simulink model "Raider_walk"  (R2016a)
settings: Solver=FixedStepAuto  StartTime=0.0  StopTime=inf  FixedStep=0.01  RelTol=1e-3
model workspace (MAT data in the model file):
  SL_ROS_VariableLengthArrays_MaxSizes.CommonInfo.ArrayTruncateAction = 'EmitWarning'
  SL_ROS_VariableLengthArrays_MaxSizes.MsgTypeMap = containers.Map
  SL_ROS_VariableLengthArrays_MaxSizes.MsgTypeMap.serialization.keys = {'sensor_msgs/JointState'}
  SL_ROS_VariableLengthArrays_MaxSizes.MsgTypeMap.serialization.values{1}(1).PropertyName = 'Name'
  SL_ROS_VariableLengthArrays_MaxSizes.MsgTypeMap.serialization.values{1}(1).DataType = 'std_msgs/String'
  SL_ROS_VariableLengthArrays_MaxSizes.MsgTypeMap.serialization.values{1}(1).MaxLength = 20
  SL_ROS_VariableLengthArrays_MaxSizes.MsgTypeMap.serialization.values{1}(2).PropertyName = 'Position'
  SL_ROS_VariableLengthArrays_MaxSizes.MsgTypeMap.serialization.values{1}(2).DataType = 'double'
  SL_ROS_VariableLengthArrays_MaxSizes.MsgTypeMap.serialization.values{1}(2).MaxLength = 128
  SL_ROS_VariableLengthArrays_MaxSizes.MsgTypeMap.serialization.values{1}(3).PropertyName = 'Velocity'
  SL_ROS_VariableLengthArrays_MaxSizes.MsgTypeMap.serialization.values{1}(3).DataType = 'double'
  SL_ROS_VariableLengthArrays_MaxSizes.MsgTypeMap.serialization.values{1}(3).MaxLength = 128
  SL_ROS_VariableLengthArrays_MaxSizes.MsgTypeMap.serialization.values{1}(4).PropertyName = 'Effort'
  SL_ROS_VariableLengthArrays_MaxSizes.MsgTypeMap.serialization.values{1}(4).DataType = 'double'
  SL_ROS_VariableLengthArrays_MaxSizes.MsgTypeMap.serialization.values{1}(4).MaxLength = 128
  SL_ROS_VariableLengthArrays_MaxSizes.MsgTypeMap.serialization.uniformity = 0
  SL_ROS_VariableLengthArrays_MaxSizes.MsgTypeMap.serialization.keyType = 'char'
  SL_ROS_VariableLengthArrays_MaxSizes.MsgTypeMap.serialization.valueType = 'any'
  currentPosition = Simulink.Signal
  currentPosition.DataType = 'double'
  currentPosition.Dimensions = [1 20]
  currentPosition.DimensionsMode = 'auto'
  currentPosition.Complexity = 'real'
  currentPosition.SampleTime = -1
  currentPosition.SamplingMode = 'auto'
  currentPosition.InitialValue = '[0 0 0 0 0 0 0 0 0 0 0 0 0 0 0 0 0 0 0 0]'
  targetPosition = Simulink.Signal
  targetPosition.DataType = 'double'
  targetPosition.Dimensions = [1 20]
  targetPosition.DimensionsMode = 'auto'
  targetPosition.Complexity = 'real'
  targetPosition.SampleTime = -1
  targetPosition.SamplingMode = 'auto'
  targetPosition.InitialValue = '[0 0 0 0 0 0 0 0 0 0 0 0 0 0 0 0 0 0 0 0]'
libraries: robotlib x81
(part 1 of 2)
settings Model: Creator=xavidz  LastModifiedBy=xavidz
settings OptimizationCC: OptimizeModelRefInitCode=on  LifeSpan=1  MaxStackSize=64
settings HardwareCC: ProdBitPerLong=64  ProdHWDeviceType=Intel->x86-64 (Linux 64)
settings RTWCC: SystemTargetFile=ert.tlc  HardwareBoard=Robot Operating System (ROS)  TemplateMakefile=ert_default_tmf  GenerateReport=on  Toolchain=Catkin  IncludeHyperlinkInReport=on  LaunchReport=on  TargetLang=C++  GenerateTraceInfo=on  GenerateTraceReport=on  GenerateTraceReportSl=on  GenerateTraceReportSf=on  GenerateTraceReportEml=on
settings CodeAppCC: ForceParamTrailComments=on  IgnoreCustomStorageClasses=off  OperatorAnnotations=on  SimulinkDataObjDesc=on  SFDataObjDesc=on  MATLABFcnDesc=on  InsertBlockDesc=on  MATLABSourceComments=on

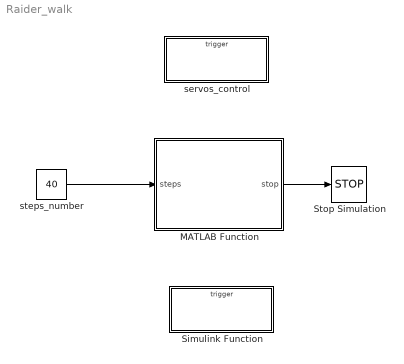
== system Raider_walk ==
  MATLAB Function : MATLAB Function  TreatAsAtomicUnit=on
  Simulink Function : Subsystem  TreatAsAtomicUnit=on
  Stop Simulation : Stop
  servos_control : Subsystem  TreatAsAtomicUnit=on
  "steps_number " : Constant  Value=40  OutDataTypeStr=uint8
  wires:
  MATLAB Function/1(stop) -> Stop Simulation/1
  "steps_number "/1 -> MATLAB Function/1(steps)

== system Raider_walk/Simulink Function ==
  delay : TriggerPort  TriggerType=function-call  IsSimulinkFunction=on  FunctionName=delay  VariantControl=Variant
  MATLAB Function : MATLAB Function  TreatAsAtomicUnit=on
  Simulink Function4 : Subsystem  TreatAsAtomicUnit=on
  t : ArgIn  DisableCoverage=on  ArgumentName=t
  wires:
  t/1 -> MATLAB Function/1(t)

== system Raider_walk/servos_control ==
  move : TriggerPort  TriggerType=function-call  IsSimulinkFunction=on  FunctionName=move  VariantControl=Variant
  MATLAB Function : MATLAB Function  TreatAsAtomicUnit=on
  Simulink Function1 : Subsystem  TreatAsAtomicUnit=on
  Simulink Function2 : Subsystem  TreatAsAtomicUnit=on
  t : ArgIn  ArgumentName=t
  wires:
  t/1 -> MATLAB Function/1(t)

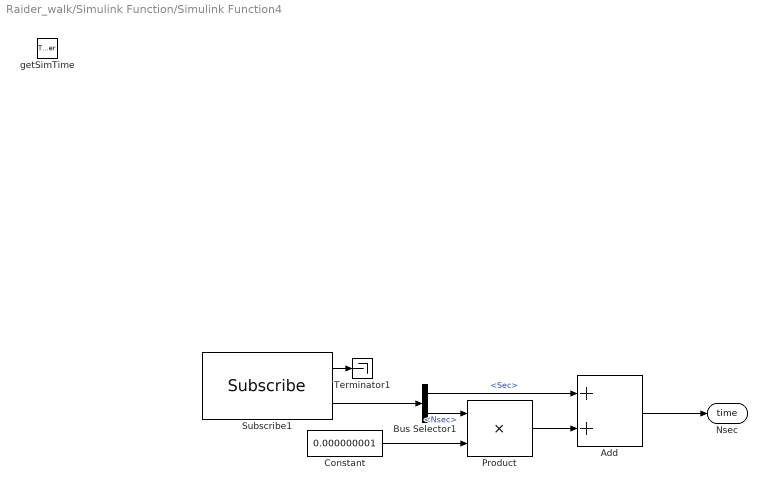
== system Raider_walk/Simulink Function/Simulink Function4 ==
  getSimTime : TriggerPort  TriggerType=function-call  IsSimulinkFunction=on  FunctionName=getSimTime  VariantControl=Variant
  Add : Sum
  Bus Selector1 : BusSelector  OutputSignals=Clock_.Sec,Clock_.Nsec
  Constant : Constant  Value=0.000000001
  Product : Product
  Subscribe1 : robotlib/Subscribe  SourceLibraryInfo=This block requires Robotics System Toolbox  topicSource=Select from ROS network  topic=/clock  messageType=rosgraph_msgs/Clock  sampleTime=-1  messageQueueLength=1
  Terminator1 : Terminator
  Nsec : ArgOut  ArgumentName=time
  wires:
  Subscribe1/2 -> Bus Selector1/1
  Bus Selector1/2 -> Product/1  "<Nsec>"
  Constant/1 -> Product/2
  Bus Selector1/1 -> Add/1  "<Sec>"
  Product/1 -> Add/2
  Add/1 -> Nsec/1
  Subscribe1/1 -> Terminator1/1

== system Raider_walk/servos_control/Simulink Function1 ==
  publishPosition : TriggerPort  TriggerType=function-call  IsSimulinkFunction=on  FunctionName=publishPosition  VariantControl=Variant
  Position_Publishers : Subsystem
  Switch Case : SwitchCase  CaseConditions={1,2,3,4,5,6,7,8,9,10,11,12,13,14,15,16,17,18,19,20}  ShowDefaultCase=off
  joint : ArgIn  DisableCoverage=on  ArgumentName=joint
  pos : ArgIn  Port=2  ArgumentName=pos
  wires:
  joint/1 -> Switch Case/1
  Switch Case/1 -> Position_Publishers/1(In1)
  Switch Case/2 -> Position_Publishers/2(In2)
  Switch Case/3 -> Position_Publishers/3(In3)
  Switch Case/4 -> Position_Publishers/4(In4)
  Switch Case/5 -> Position_Publishers/5(In5)
  Switch Case/6 -> Position_Publishers/6(In6)
  pos/1 -> Position_Publishers/21("In21 ")
  Switch Case/20 -> Position_Publishers/20(In20)
  Switch Case/19 -> Position_Publishers/19(In19)
  Switch Case/18 -> Position_Publishers/18(In18)
  Switch Case/16 -> Position_Publishers/16(In16)
  Switch Case/17 -> Position_Publishers/17(In17)
  Switch Case/15 -> Position_Publishers/15(In15)
  Switch Case/14 -> Position_Publishers/14(In14)
  Switch Case/13 -> Position_Publishers/13(In13)
  Switch Case/12 -> Position_Publishers/12(In12)
  Switch Case/11 -> Position_Publishers/11(In11)
  Switch Case/10 -> Position_Publishers/10(In10)
  Switch Case/9 -> Position_Publishers/9(In9)
  Switch Case/8 -> Position_Publishers/8(In8)
  Switch Case/7 -> Position_Publishers/7(In7)

== system Raider_walk/servos_control/Simulink Function2 ==
  publishVelocity : TriggerPort  TriggerType=function-call  IsSimulinkFunction=on  FunctionName=publishVelocity  VariantControl=Variant
  Switch Case : SwitchCase  CaseConditions={1,2,3,4,5,6,7,8,9,10,11,12,13,14,15,16,17,18,19,20}  ShowDefaultCase=off
  Velocity_Publishers : Subsystem
  joint : ArgIn  DisableCoverage=on  ArgumentName=joint
  vel : ArgIn  Port=2  ArgumentName=vel
  wires:
  joint/1 -> Switch Case/1
  Switch Case/1 -> Velocity_Publishers/1(In1)
  Switch Case/2 -> Velocity_Publishers/2(In2)
  Switch Case/3 -> Velocity_Publishers/3(In3)
  Switch Case/4 -> Velocity_Publishers/4(In4)
  Switch Case/5 -> Velocity_Publishers/5(In5)
  Switch Case/6 -> Velocity_Publishers/6(In6)
  vel/1 -> Velocity_Publishers/21("In21 ")
  Switch Case/20 -> Velocity_Publishers/20(In20)
  Switch Case/19 -> Velocity_Publishers/19(In19)
  Switch Case/18 -> Velocity_Publishers/18(In18)
  Switch Case/16 -> Velocity_Publishers/16(In16)
  Switch Case/17 -> Velocity_Publishers/17(In17)
  Switch Case/15 -> Velocity_Publishers/15(In15)
  Switch Case/14 -> Velocity_Publishers/14(In14)
  Switch Case/13 -> Velocity_Publishers/13(In13)
  Switch Case/12 -> Velocity_Publishers/12(In12)
  Switch Case/11 -> Velocity_Publishers/11(In11)
  Switch Case/10 -> Velocity_Publishers/10(In10)
  Switch Case/9 -> Velocity_Publishers/9(In9)
  Switch Case/8 -> Velocity_Publishers/8(In8)
  Switch Case/7 -> Velocity_Publishers/7(In7)

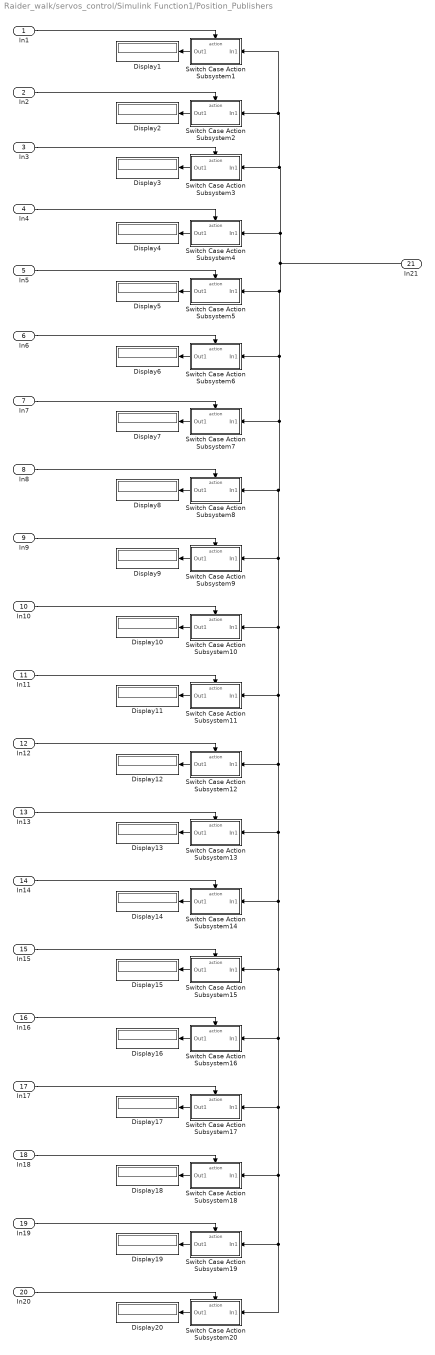
== system Raider_walk/servos_control/Simulink Function1/Position_Publishers ==
  In1 : Inport
  In2 : Inport  Port=2
  In3 : Inport  Port=3
  In4 : Inport  Port=4
  In5 : Inport  Port=5
  In6 : Inport  Port=6
  In7 : Inport  Port=7
  In8 : Inport  Port=8
  In9 : Inport  Port=9
  In10 : Inport  Port=10
  In11 : Inport  Port=11
  In12 : Inport  Port=12
  In13 : Inport  Port=13
  In14 : Inport  Port=14
  In15 : Inport  Port=15
  In16 : Inport  Port=16
  In17 : Inport  Port=17
  In18 : Inport  Port=18
  In19 : Inport  Port=19
  In20 : Inport  Port=20
  "In21 " : Inport  Port=21
  Display{1..20} (20 alike) : Display
  "Switch Case Action Subsystem1 " : Subsystem  TreatAsAtomicUnit=on
  Switch Case Action Subsystem10 : Subsystem  TreatAsAtomicUnit=on
  Switch Case Action Subsystem11 : Subsystem  TreatAsAtomicUnit=on
  Switch Case Action Subsystem12 : Subsystem  TreatAsAtomicUnit=on
  Switch Case Action Subsystem13 : Subsystem  TreatAsAtomicUnit=on
  Switch Case Action Subsystem14 : Subsystem  TreatAsAtomicUnit=on
  Switch Case Action Subsystem15 : Subsystem  TreatAsAtomicUnit=on
  Switch Case Action Subsystem16 : Subsystem  TreatAsAtomicUnit=on
  Switch Case Action Subsystem17 : Subsystem  TreatAsAtomicUnit=on
  Switch Case Action Subsystem18 : Subsystem  TreatAsAtomicUnit=on
  Switch Case Action Subsystem19 : Subsystem  TreatAsAtomicUnit=on
  "Switch Case Action Subsystem2 " : Subsystem  TreatAsAtomicUnit=on
  Switch Case Action Subsystem20 : Subsystem  TreatAsAtomicUnit=on
  "Switch Case Action Subsystem3 " : Subsystem  TreatAsAtomicUnit=on
  "Switch Case Action Subsystem4 " : Subsystem  TreatAsAtomicUnit=on
  "Switch Case Action Subsystem5 " : Subsystem  TreatAsAtomicUnit=on
  "Switch Case Action Subsystem6 " : Subsystem  TreatAsAtomicUnit=on
  Switch Case Action Subsystem7 : Subsystem  TreatAsAtomicUnit=on
  Switch Case Action Subsystem8 : Subsystem  TreatAsAtomicUnit=on
  Switch Case Action Subsystem9 : Subsystem  TreatAsAtomicUnit=on
  wires:
  "In21 "/1 -> "Switch Case Action Subsystem1 "/1(In1), "Switch Case Action Subsystem2 "/1(In1), "Switch Case Action Subsystem3 "/1(In1), "Switch Case Action Subsystem4 "/1(In1), Switch Case Action Subsystem20/1(In1), Switch Case Action Subsystem19/1(In1), Switch Case Action Subsystem18/1(In1), Switch Case Action Subsystem17/1(In1), Switch Case Action Subsystem16/1(In1), Switch Case Action Subsystem15/1(In1), Switch Case Action Subsystem14/1(In1), Switch Case Action Subsystem13/1(In1), Switch Case Action Subsystem12/1(In1), Switch Case Action Subsystem11/1(In1), Switch Case Action Subsystem10/1(In1), Switch Case Action Subsystem9/1(In1), Switch Case Action Subsystem8/1(In1), Switch Case Action Subsystem7/1(In1), "Switch Case Action Subsystem6 "/1(In1), "Switch Case Action Subsystem5 "/1(In1)
  In1/1 -> "Switch Case Action Subsystem1 "/Action
  In6/1 -> "Switch Case Action Subsystem6 "/Action
  In3/1 -> "Switch Case Action Subsystem3 "/Action
  "Switch Case Action Subsystem5 "/1(Out1) -> Display5/1
  "Switch Case Action Subsystem3 "/1(Out1) -> Display3/1
  "Switch Case Action Subsystem2 "/1(Out1) -> Display2/1
  In4/1 -> "Switch Case Action Subsystem4 "/Action
  "Switch Case Action Subsystem6 "/1(Out1) -> Display6/1
  "Switch Case Action Subsystem1 "/1(Out1) -> Display1/1
  In2/1 -> "Switch Case Action Subsystem2 "/Action
  "Switch Case Action Subsystem4 "/1(Out1) -> Display4/1
  In5/1 -> "Switch Case Action Subsystem5 "/Action
  In7/1 -> Switch Case Action Subsystem7/Action
  Switch Case Action Subsystem7/1(Out1) -> Display7/1
  In8/1 -> Switch Case Action Subsystem8/Action
  Switch Case Action Subsystem8/1(Out1) -> Display8/1
  In9/1 -> Switch Case Action Subsystem9/Action
  Switch Case Action Subsystem9/1(Out1) -> Display9/1
  In10/1 -> Switch Case Action Subsystem10/Action
  Switch Case Action Subsystem10/1(Out1) -> Display10/1
  In11/1 -> Switch Case Action Subsystem11/Action
  Switch Case Action Subsystem11/1(Out1) -> Display11/1
  In12/1 -> Switch Case Action Subsystem12/Action
  Switch Case Action Subsystem12/1(Out1) -> Display12/1
  In13/1 -> Switch Case Action Subsystem13/Action
  Switch Case Action Subsystem13/1(Out1) -> Display13/1
  In14/1 -> Switch Case Action Subsystem14/Action
  Switch Case Action Subsystem14/1(Out1) -> Display14/1
  In15/1 -> Switch Case Action Subsystem15/Action
  Switch Case Action Subsystem15/1(Out1) -> Display15/1
  In16/1 -> Switch Case Action Subsystem16/Action
  Switch Case Action Subsystem16/1(Out1) -> Display16/1
  In17/1 -> Switch Case Action Subsystem17/Action
  Switch Case Action Subsystem17/1(Out1) -> Display17/1
  In18/1 -> Switch Case Action Subsystem18/Action
  Switch Case Action Subsystem18/1(Out1) -> Display18/1
  In19/1 -> Switch Case Action Subsystem19/Action
  Switch Case Action Subsystem19/1(Out1) -> Display19/1
  In20/1 -> Switch Case Action Subsystem20/Action
  Switch Case Action Subsystem20/1(Out1) -> Display20/1

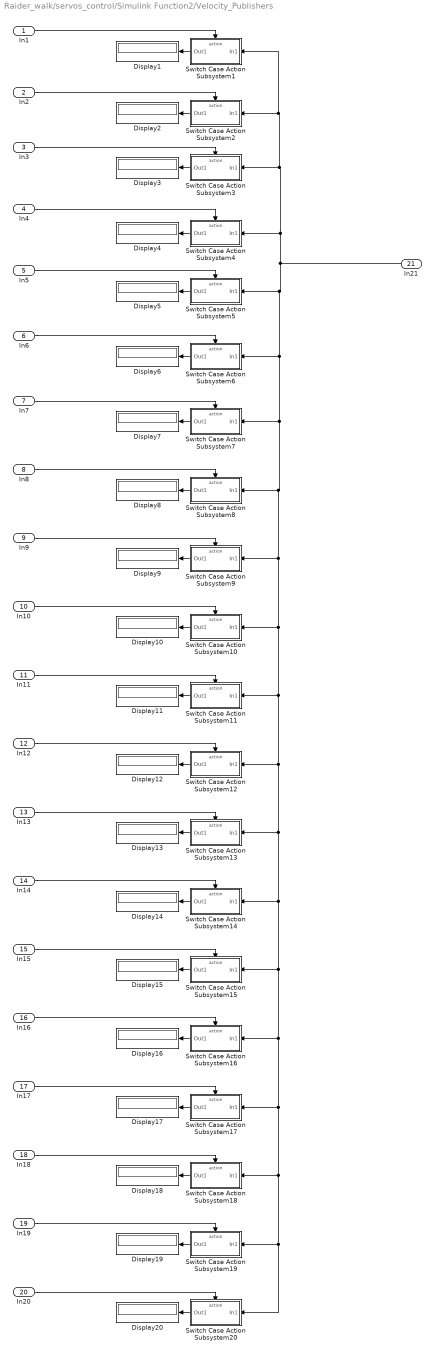
== system Raider_walk/servos_control/Simulink Function2/Velocity_Publishers ==
  In1 : Inport
  In2 : Inport  Port=2
  In3 : Inport  Port=3
  In4 : Inport  Port=4
  In5 : Inport  Port=5
  In6 : Inport  Port=6
  In7 : Inport  Port=7
  In8 : Inport  Port=8
  In9 : Inport  Port=9
  In10 : Inport  Port=10
  In11 : Inport  Port=11
  In12 : Inport  Port=12
  In13 : Inport  Port=13
  In14 : Inport  Port=14
  In15 : Inport  Port=15
  In16 : Inport  Port=16
  In17 : Inport  Port=17
  In18 : Inport  Port=18
  In19 : Inport  Port=19
  In20 : Inport  Port=20
  "In21 " : Inport  Port=21
  Display{1..20} (20 alike) : Display
  "Switch Case Action Subsystem1 " : Subsystem  TreatAsAtomicUnit=on
  Switch Case Action Subsystem10 : Subsystem  TreatAsAtomicUnit=on
  Switch Case Action Subsystem11 : Subsystem  TreatAsAtomicUnit=on
  Switch Case Action Subsystem12 : Subsystem  TreatAsAtomicUnit=on
  Switch Case Action Subsystem13 : Subsystem  TreatAsAtomicUnit=on
  Switch Case Action Subsystem14 : Subsystem  TreatAsAtomicUnit=on
  Switch Case Action Subsystem15 : Subsystem  TreatAsAtomicUnit=on
  Switch Case Action Subsystem16 : Subsystem  TreatAsAtomicUnit=on
  Switch Case Action Subsystem17 : Subsystem  TreatAsAtomicUnit=on
  Switch Case Action Subsystem18 : Subsystem  TreatAsAtomicUnit=on
  Switch Case Action Subsystem19 : Subsystem  TreatAsAtomicUnit=on
  "Switch Case Action Subsystem2 " : Subsystem  TreatAsAtomicUnit=on
  Switch Case Action Subsystem20 : Subsystem  TreatAsAtomicUnit=on
  "Switch Case Action Subsystem3 " : Subsystem  TreatAsAtomicUnit=on
  "Switch Case Action Subsystem4 " : Subsystem  TreatAsAtomicUnit=on
  "Switch Case Action Subsystem5 " : Subsystem  TreatAsAtomicUnit=on
  "Switch Case Action Subsystem6 " : Subsystem  TreatAsAtomicUnit=on
  Switch Case Action Subsystem7 : Subsystem  TreatAsAtomicUnit=on
  Switch Case Action Subsystem8 : Subsystem  TreatAsAtomicUnit=on
  Switch Case Action Subsystem9 : Subsystem  TreatAsAtomicUnit=on
  wires:
  "In21 "/1 -> "Switch Case Action Subsystem1 "/1(In1), "Switch Case Action Subsystem2 "/1(In1), "Switch Case Action Subsystem3 "/1(In1), "Switch Case Action Subsystem4 "/1(In1), Switch Case Action Subsystem20/1(In1), Switch Case Action Subsystem19/1(In1), Switch Case Action Subsystem18/1(In1), Switch Case Action Subsystem17/1(In1), Switch Case Action Subsystem16/1(In1), Switch Case Action Subsystem15/1(In1), Switch Case Action Subsystem14/1(In1), Switch Case Action Subsystem13/1(In1), Switch Case Action Subsystem12/1(In1), Switch Case Action Subsystem11/1(In1), Switch Case Action Subsystem10/1(In1), Switch Case Action Subsystem9/1(In1), Switch Case Action Subsystem8/1(In1), Switch Case Action Subsystem7/1(In1), "Switch Case Action Subsystem6 "/1(In1), "Switch Case Action Subsystem5 "/1(In1)
  In1/1 -> "Switch Case Action Subsystem1 "/Action
  In6/1 -> "Switch Case Action Subsystem6 "/Action
  In3/1 -> "Switch Case Action Subsystem3 "/Action
  "Switch Case Action Subsystem5 "/1(Out1) -> Display5/1
  "Switch Case Action Subsystem3 "/1(Out1) -> Display3/1
  "Switch Case Action Subsystem2 "/1(Out1) -> Display2/1
  In4/1 -> "Switch Case Action Subsystem4 "/Action
  "Switch Case Action Subsystem6 "/1(Out1) -> Display6/1
  "Switch Case Action Subsystem1 "/1(Out1) -> Display1/1
  In2/1 -> "Switch Case Action Subsystem2 "/Action
  "Switch Case Action Subsystem4 "/1(Out1) -> Display4/1
  In5/1 -> "Switch Case Action Subsystem5 "/Action
  In7/1 -> Switch Case Action Subsystem7/Action
  Switch Case Action Subsystem7/1(Out1) -> Display7/1
  In8/1 -> Switch Case Action Subsystem8/Action
  Switch Case Action Subsystem8/1(Out1) -> Display8/1
  In9/1 -> Switch Case Action Subsystem9/Action
  Switch Case Action Subsystem9/1(Out1) -> Display9/1
  In10/1 -> Switch Case Action Subsystem10/Action
  Switch Case Action Subsystem10/1(Out1) -> Display10/1
  In11/1 -> Switch Case Action Subsystem11/Action
  Switch Case Action Subsystem11/1(Out1) -> Display11/1
  In12/1 -> Switch Case Action Subsystem12/Action
  Switch Case Action Subsystem12/1(Out1) -> Display12/1
  In13/1 -> Switch Case Action Subsystem13/Action
  Switch Case Action Subsystem13/1(Out1) -> Display13/1
  In14/1 -> Switch Case Action Subsystem14/Action
  Switch Case Action Subsystem14/1(Out1) -> Display14/1
  In15/1 -> Switch Case Action Subsystem15/Action
  Switch Case Action Subsystem15/1(Out1) -> Display15/1
  In16/1 -> Switch Case Action Subsystem16/Action
  Switch Case Action Subsystem16/1(Out1) -> Display16/1
  In17/1 -> Switch Case Action Subsystem17/Action
  Switch Case Action Subsystem17/1(Out1) -> Display17/1
  In18/1 -> Switch Case Action Subsystem18/Action
  Switch Case Action Subsystem18/1(Out1) -> Display18/1
  In19/1 -> Switch Case Action Subsystem19/Action
  Switch Case Action Subsystem19/1(Out1) -> Display19/1
  In20/1 -> Switch Case Action Subsystem20/Action
  Switch Case Action Subsystem20/1(Out1) -> Display20/1

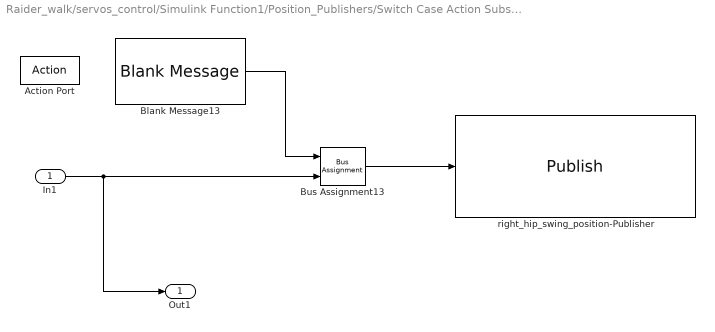
== system Raider_walk/servos_control/Simulink Function1/Position_Publishers/Switch Case Action Subsystem1  ==
  In1 : Inport
  Action Port : ActionPort  ActionType=case
  Blank Message13 : robotlib/Blank Message  SourceLibraryInfo=This block requires Robotics System Toolbox  messageType=std_msgs/Float64  SampleTime=inf
  Bus Assignment13 : BusAssignment  AssignedSignals=Data
  right_hip_swing_position-Publisher : robotlib/Publish  SourceLibraryInfo=This block requires Robotics System Toolbox  topicSource=Select from ROS network  topic=/raider/middle_hip_twist_position_controller/command  messageType=std_msgs/Float64  messageQueueLength=1
  Out1 : Outport
  wires:
  Blank Message13/1 -> Bus Assignment13/1
  Bus Assignment13/1 -> right_hip_swing_position-Publisher/1
  In1/1 -> Out1/1, Bus Assignment13/2

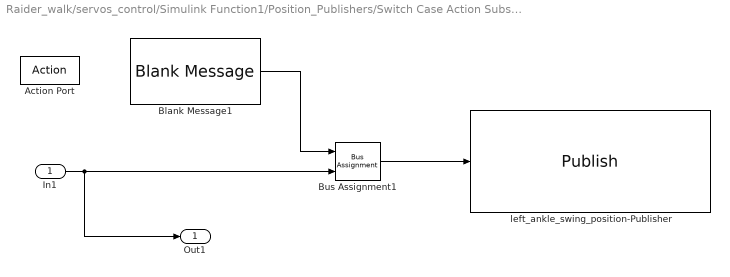
== system Raider_walk/servos_control/Simulink Function1/Position_Publishers/Switch Case Action Subsystem10 ==
  In1 : Inport
  Action Port : ActionPort  ActionType=case
  Blank Message1 : robotlib/Blank Message  SourceLibraryInfo=This block requires Robotics System Toolbox  messageType=std_msgs/Float64  SampleTime=inf
  Bus Assignment1 : BusAssignment  AssignedSignals=Data
  left_ankle_swing_position-Publisher : robotlib/Publish  SourceLibraryInfo=This block requires Robotics System Toolbox  topicSource=Select from ROS network  topic=/raider/l_hip_twist_position_controller/command  messageType=std_msgs/Float64  messageQueueLength=1
  Out1 : Outport
  wires:
  Blank Message1/1 -> Bus Assignment1/1
  Bus Assignment1/1 -> left_ankle_swing_position-Publisher/1
  In1/1 -> Out1/1, Bus Assignment1/2

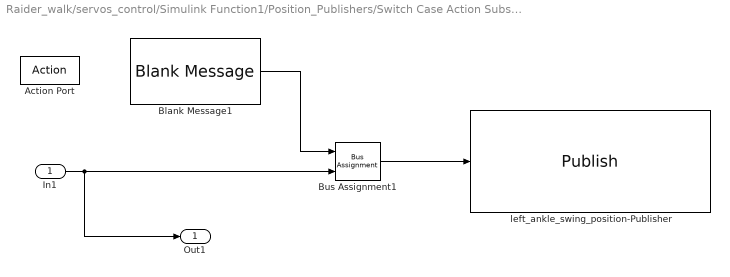
== system Raider_walk/servos_control/Simulink Function1/Position_Publishers/Switch Case Action Subsystem11 ==
  In1 : Inport
  Action Port : ActionPort  ActionType=case
  Blank Message1 : robotlib/Blank Message  SourceLibraryInfo=This block requires Robotics System Toolbox  messageType=std_msgs/Float64  SampleTime=inf
  Bus Assignment1 : BusAssignment  AssignedSignals=Data
  left_ankle_swing_position-Publisher : robotlib/Publish  SourceLibraryInfo=This block requires Robotics System Toolbox  topicSource=Select from ROS network  topic=/raider/r_hip_lateral_position_controller/command  messageType=std_msgs/Float64  messageQueueLength=1
  Out1 : Outport
  wires:
  Blank Message1/1 -> Bus Assignment1/1
  Bus Assignment1/1 -> left_ankle_swing_position-Publisher/1
  In1/1 -> Out1/1, Bus Assignment1/2

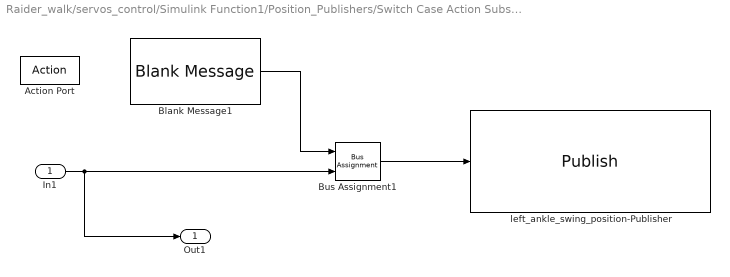
== system Raider_walk/servos_control/Simulink Function1/Position_Publishers/Switch Case Action Subsystem12 ==
  In1 : Inport
  Action Port : ActionPort  ActionType=case
  Blank Message1 : robotlib/Blank Message  SourceLibraryInfo=This block requires Robotics System Toolbox  messageType=std_msgs/Float64  SampleTime=inf
  Bus Assignment1 : BusAssignment  AssignedSignals=Data
  left_ankle_swing_position-Publisher : robotlib/Publish  SourceLibraryInfo=This block requires Robotics System Toolbox  topicSource=Select from ROS network  topic=/raider/l_hip_lateral_position_controller/command  messageType=std_msgs/Float64  messageQueueLength=1
  Out1 : Outport
  wires:
  Blank Message1/1 -> Bus Assignment1/1
  Bus Assignment1/1 -> left_ankle_swing_position-Publisher/1
  In1/1 -> Out1/1, Bus Assignment1/2

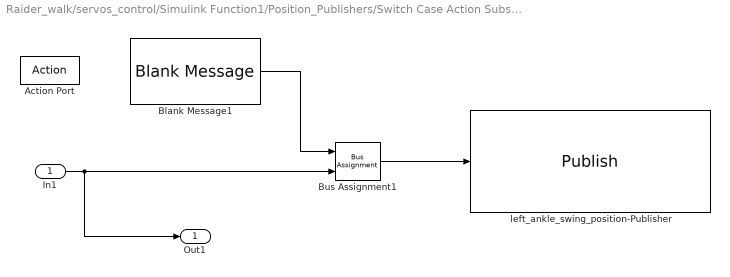
== system Raider_walk/servos_control/Simulink Function1/Position_Publishers/Switch Case Action Subsystem13 ==
  In1 : Inport
  Action Port : ActionPort  ActionType=case
  Blank Message1 : robotlib/Blank Message  SourceLibraryInfo=This block requires Robotics System Toolbox  messageType=std_msgs/Float64  SampleTime=inf
  Bus Assignment1 : BusAssignment  AssignedSignals=Data
  left_ankle_swing_position-Publisher : robotlib/Publish  SourceLibraryInfo=This block requires Robotics System Toolbox  topicSource=Select from ROS network  topic=/raider/r_hip_swing_position_controller/command  messageType=std_msgs/Float64  messageQueueLength=1
  Out1 : Outport
  wires:
  Blank Message1/1 -> Bus Assignment1/1
  Bus Assignment1/1 -> left_ankle_swing_position-Publisher/1
  In1/1 -> Out1/1, Bus Assignment1/2

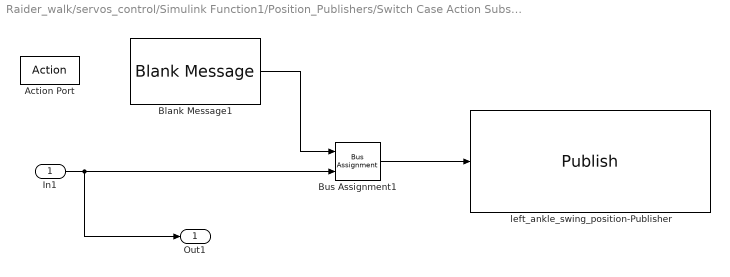
== system Raider_walk/servos_control/Simulink Function1/Position_Publishers/Switch Case Action Subsystem14 ==
  In1 : Inport
  Action Port : ActionPort  ActionType=case
  Blank Message1 : robotlib/Blank Message  SourceLibraryInfo=This block requires Robotics System Toolbox  messageType=std_msgs/Float64  SampleTime=inf
  Bus Assignment1 : BusAssignment  AssignedSignals=Data
  left_ankle_swing_position-Publisher : robotlib/Publish  SourceLibraryInfo=This block requires Robotics System Toolbox  topicSource=Select from ROS network  topic=/raider/l_hip_swing_position_controller/command  messageType=std_msgs/Float64  messageQueueLength=1
  Out1 : Outport
  wires:
  Blank Message1/1 -> Bus Assignment1/1
  Bus Assignment1/1 -> left_ankle_swing_position-Publisher/1
  In1/1 -> Out1/1, Bus Assignment1/2

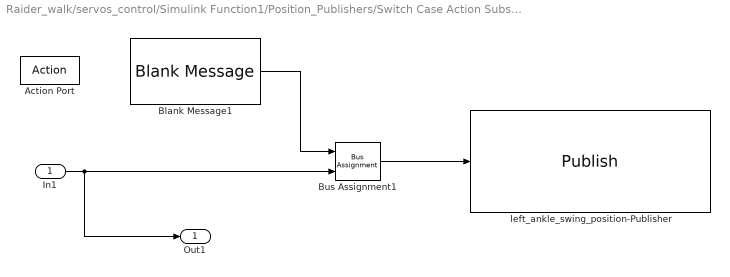
== system Raider_walk/servos_control/Simulink Function1/Position_Publishers/Switch Case Action Subsystem15 ==
  In1 : Inport
  Action Port : ActionPort  ActionType=case
  Blank Message1 : robotlib/Blank Message  SourceLibraryInfo=This block requires Robotics System Toolbox  messageType=std_msgs/Float64  SampleTime=inf
  Bus Assignment1 : BusAssignment  AssignedSignals=Data
  left_ankle_swing_position-Publisher : robotlib/Publish  SourceLibraryInfo=This block requires Robotics System Toolbox  topicSource=Select from ROS network  topic=/raider/r_upper_knee_position_controller/command  messageType=std_msgs/Float64  messageQueueLength=1
  Out1 : Outport
  wires:
  Blank Message1/1 -> Bus Assignment1/1
  Bus Assignment1/1 -> left_ankle_swing_position-Publisher/1
  In1/1 -> Out1/1, Bus Assignment1/2

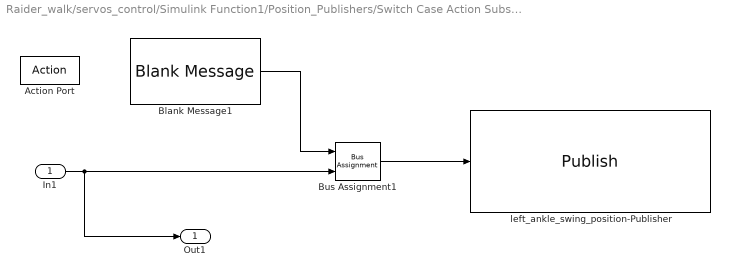
== system Raider_walk/servos_control/Simulink Function1/Position_Publishers/Switch Case Action Subsystem16 ==
  In1 : Inport
  Action Port : ActionPort  ActionType=case
  Blank Message1 : robotlib/Blank Message  SourceLibraryInfo=This block requires Robotics System Toolbox  messageType=std_msgs/Float64  SampleTime=inf
  Bus Assignment1 : BusAssignment  AssignedSignals=Data
  left_ankle_swing_position-Publisher : robotlib/Publish  SourceLibraryInfo=This block requires Robotics System Toolbox  topicSource=Select from ROS network  topic=/raider/l_upper_knee_position_controller/command  messageType=std_msgs/Float64  messageQueueLength=1
  Out1 : Outport
  wires:
  Blank Message1/1 -> Bus Assignment1/1
  Bus Assignment1/1 -> left_ankle_swing_position-Publisher/1
  In1/1 -> Out1/1, Bus Assignment1/2

== system Raider_walk/servos_control/Simulink Function1/Position_Publishers/Switch Case Action Subsystem17 ==
  In1 : Inport
  Action Port : ActionPort  ActionType=case
  Blank Message1 : robotlib/Blank Message  SourceLibraryInfo=This block requires Robotics System Toolbox  messageType=std_msgs/Float64  SampleTime=inf
  Bus Assignment1 : BusAssignment  AssignedSignals=Data
  left_ankle_swing_position-Publisher : robotlib/Publish  SourceLibraryInfo=This block requires Robotics System Toolbox  topicSource=Select from ROS network  topic=/raider/r_ankle_swing_position_controller/command  messageType=std_msgs/Float64  messageQueueLength=1
  Out1 : Outport
  wires:
  Blank Message1/1 -> Bus Assignment1/1
  Bus Assignment1/1 -> left_ankle_swing_position-Publisher/1
  In1/1 -> Out1/1, Bus Assignment1/2

== system Raider_walk/servos_control/Simulink Function1/Position_Publishers/Switch Case Action Subsystem18 ==
  In1 : Inport
  Action Port : ActionPort  ActionType=case
  Blank Message1 : robotlib/Blank Message  SourceLibraryInfo=This block requires Robotics System Toolbox  messageType=std_msgs/Float64  SampleTime=inf
  Bus Assignment1 : BusAssignment  AssignedSignals=Data
  left_ankle_swing_position-Publisher : robotlib/Publish  SourceLibraryInfo=This block requires Robotics System Toolbox  topicSource=Select from ROS network  topic=/raider/l_ankle_swing_position_controller/command  messageType=std_msgs/Float64  messageQueueLength=1
  Out1 : Outport
  wires:
  Blank Message1/1 -> Bus Assignment1/1
  Bus Assignment1/1 -> left_ankle_swing_position-Publisher/1
  In1/1 -> Out1/1, Bus Assignment1/2

== system Raider_walk/servos_control/Simulink Function1/Position_Publishers/Switch Case Action Subsystem19 ==
  In1 : Inport
  Action Port : ActionPort  ActionType=case
  Blank Message1 : robotlib/Blank Message  SourceLibraryInfo=This block requires Robotics System Toolbox  messageType=std_msgs/Float64  SampleTime=inf
  Bus Assignment1 : BusAssignment  AssignedSignals=Data
  left_ankle_swing_position-Publisher : robotlib/Publish  SourceLibraryInfo=This block requires Robotics System Toolbox  topicSource=Select from ROS network  topic=/raider/r_ankle_lateral_position_controller/command  messageType=std_msgs/Float64  messageQueueLength=1
  Out1 : Outport
  wires:
  Blank Message1/1 -> Bus Assignment1/1
  Bus Assignment1/1 -> left_ankle_swing_position-Publisher/1
  In1/1 -> Out1/1, Bus Assignment1/2

== system Raider_walk/servos_control/Simulink Function1/Position_Publishers/Switch Case Action Subsystem2  ==
  In1 : Inport
  Action Port : ActionPort  ActionType=case
  Blank Message4 : robotlib/Blank Message  SourceLibraryInfo=This block requires Robotics System Toolbox  messageType=std_msgs/Float64  SampleTime=inf
  Bus Assignment4 : BusAssignment  AssignedSignals=Data
  left_hip_swing_position-Publisher : robotlib/Publish  SourceLibraryInfo=This block requires Robotics System Toolbox  topicSource=Select from ROS network  topic=/raider/neck_position_controller/command  messageType=std_msgs/Float64  messageQueueLength=1
  Out1 : Outport
  wires:
  Blank Message4/1 -> Bus Assignment4/1
  Bus Assignment4/1 -> left_hip_swing_position-Publisher/1
  In1/1 -> Out1/1, Bus Assignment4/2

== system Raider_walk/servos_control/Simulink Function1/Position_Publishers/Switch Case Action Subsystem20 ==
  In1 : Inport
  Action Port : ActionPort  ActionType=case
  Blank Message1 : robotlib/Blank Message  SourceLibraryInfo=This block requires Robotics System Toolbox  messageType=std_msgs/Float64  SampleTime=inf
  Bus Assignment1 : BusAssignment  AssignedSignals=Data
  left_ankle_swing_position-Publisher : robotlib/Publish  SourceLibraryInfo=This block requires Robotics System Toolbox  topicSource=Select from ROS network  topic=/raider/l_ankle_lateral_position_controller/command  messageType=std_msgs/Float64  messageQueueLength=1
  Out1 : Outport
  wires:
  Blank Message1/1 -> Bus Assignment1/1
  Bus Assignment1/1 -> left_ankle_swing_position-Publisher/1
  In1/1 -> Out1/1, Bus Assignment1/2

== system Raider_walk/servos_control/Simulink Function1/Position_Publishers/Switch Case Action Subsystem3  ==
  In1 : Inport
  Action Port : ActionPort  ActionType=case
  Blank Message40 : robotlib/Blank Message  SourceLibraryInfo=This block requires Robotics System Toolbox  messageType=std_msgs/Float64  SampleTime=inf
  Bus Assignment40 : BusAssignment  AssignedSignals=Data
  right_upper_knee_position-Publisher : robotlib/Publish  SourceLibraryInfo=This block requires Robotics System Toolbox  topicSource=Select from ROS network  topic=/raider/r_shoulder_swing_position_controller/command  messageType=std_msgs/Float64  messageQueueLength=1
  Out1 : Outport
  wires:
  Blank Message40/1 -> Bus Assignment40/1
  Bus Assignment40/1 -> right_upper_knee_position-Publisher/1
  In1/1 -> Out1/1, Bus Assignment40/2

== system Raider_walk/servos_control/Simulink Function1/Position_Publishers/Switch Case Action Subsystem4  ==
  In1 : Inport
  Action Port : ActionPort  ActionType=case
  Blank Message29 : robotlib/Blank Message  SourceLibraryInfo=This block requires Robotics System Toolbox  messageType=std_msgs/Float64  SampleTime=inf
  Bus Assignment29 : BusAssignment  AssignedSignals=Data
  left_upper_knee_position-Publisher : robotlib/Publish  SourceLibraryInfo=This block requires Robotics System Toolbox  topicSource=Select from ROS network  topic=/raider/l_shoulder_swing_position_controller/command  messageType=std_msgs/Float64  messageQueueLength=1
  Out1 : Outport
  wires:
  Blank Message29/1 -> Bus Assignment29/1
  Bus Assignment29/1 -> left_upper_knee_position-Publisher/1
  In1/1 -> Out1/1, Bus Assignment29/2

== system Raider_walk/servos_control/Simulink Function1/Position_Publishers/Switch Case Action Subsystem5  ==
  In1 : Inport
  Action Port : ActionPort  ActionType=case
  Blank Message10 : robotlib/Blank Message  SourceLibraryInfo=This block requires Robotics System Toolbox  messageType=std_msgs/Float64  SampleTime=inf
  Bus Assignment10 : BusAssignment  AssignedSignals=Data
  right_ankle-swing-Publisher : robotlib/Publish  SourceLibraryInfo=This block requires Robotics System Toolbox  topicSource=Select from ROS network  topic=/raider/r_shoulder_lateral_position_controller/command  messageType=std_msgs/Float64  messageQueueLength=1
  Out1 : Outport
  wires:
  Blank Message10/1 -> Bus Assignment10/1
  Bus Assignment10/1 -> right_ankle-swing-Publisher/1
  In1/1 -> Out1/1, Bus Assignment10/2

== system Raider_walk/servos_control/Simulink Function1/Position_Publishers/Switch Case Action Subsystem6  ==
  In1 : Inport
  Action Port : ActionPort  ActionType=case
  Blank Message1 : robotlib/Blank Message  SourceLibraryInfo=This block requires Robotics System Toolbox  messageType=std_msgs/Float64  SampleTime=inf
  Bus Assignment1 : BusAssignment  AssignedSignals=Data
  left_ankle_swing_position-Publisher : robotlib/Publish  SourceLibraryInfo=This block requires Robotics System Toolbox  topicSource=Select from ROS network  topic=/raider/l_shoulder_lateral_position_controller/command  messageType=std_msgs/Float64  messageQueueLength=1
  Out1 : Outport
  wires:
  In1/1 -> Out1/1, Bus Assignment1/2
  Blank Message1/1 -> Bus Assignment1/1
  Bus Assignment1/1 -> left_ankle_swing_position-Publisher/1

== system Raider_walk/servos_control/Simulink Function1/Position_Publishers/Switch Case Action Subsystem7 ==
  In1 : Inport
  Action Port : ActionPort  ActionType=case
  Blank Message1 : robotlib/Blank Message  SourceLibraryInfo=This block requires Robotics System Toolbox  messageType=std_msgs/Float64  SampleTime=inf
  Bus Assignment1 : BusAssignment  AssignedSignals=Data
  left_ankle_swing_position-Publisher : robotlib/Publish  SourceLibraryInfo=This block requires Robotics System Toolbox  topicSource=Select from ROS network  topic=/raider/r_elbow_position_controller/command  messageType=std_msgs/Float64  messageQueueLength=1
  Out1 : Outport
  wires:
  Blank Message1/1 -> Bus Assignment1/1
  Bus Assignment1/1 -> left_ankle_swing_position-Publisher/1
  In1/1 -> Out1/1, Bus Assignment1/2

== system Raider_walk/servos_control/Simulink Function1/Position_Publishers/Switch Case Action Subsystem8 ==
  In1 : Inport
  Action Port : ActionPort  ActionType=case
  Blank Message1 : robotlib/Blank Message  SourceLibraryInfo=This block requires Robotics System Toolbox  messageType=std_msgs/Float64  SampleTime=inf
  Bus Assignment1 : BusAssignment  AssignedSignals=Data
  left_ankle_swing_position-Publisher : robotlib/Publish  SourceLibraryInfo=This block requires Robotics System Toolbox  topicSource=Select from ROS network  topic=/raider/l_elbow_position_controller/command  messageType=std_msgs/Float64  messageQueueLength=1
  Out1 : Outport
  wires:
  Blank Message1/1 -> Bus Assignment1/1
  Bus Assignment1/1 -> left_ankle_swing_position-Publisher/1
  In1/1 -> Out1/1, Bus Assignment1/2

== system Raider_walk/servos_control/Simulink Function1/Position_Publishers/Switch Case Action Subsystem9 ==
  In1 : Inport
  Action Port : ActionPort  ActionType=case
  Blank Message1 : robotlib/Blank Message  SourceLibraryInfo=This block requires Robotics System Toolbox  messageType=std_msgs/Float64  SampleTime=inf
  Bus Assignment1 : BusAssignment  AssignedSignals=Data
  left_ankle_swing_position-Publisher : robotlib/Publish  SourceLibraryInfo=This block requires Robotics System Toolbox  topicSource=Select from ROS network  topic=/raider/l_hip_twist_position_controller/command  messageType=std_msgs/Float64  messageQueueLength=1
  Out1 : Outport
  wires:
  Blank Message1/1 -> Bus Assignment1/1
  Bus Assignment1/1 -> left_ankle_swing_position-Publisher/1
  In1/1 -> Out1/1, Bus Assignment1/2

== system Raider_walk/servos_control/Simulink Function2/Velocity_Publishers/Switch Case Action Subsystem1  ==
  In1 : Inport
  Action Port : ActionPort  ActionType=case
  Blank Message13 : robotlib/Blank Message  SourceLibraryInfo=This block requires Robotics System Toolbox  messageType=std_msgs/Float64  SampleTime=inf
  Bus Assignment13 : BusAssignment  AssignedSignals=Data
  right_hip_swing_position-Publisher : robotlib/Publish  SourceLibraryInfo=This block requires Robotics System Toolbox  topicSource=Select from ROS network  topic=/raider/middle_hip_twist_velocity_controller/command  messageType=std_msgs/Float64  messageQueueLength=1
  Out1 : Outport
  wires:
  Blank Message13/1 -> Bus Assignment13/1
  Bus Assignment13/1 -> right_hip_swing_position-Publisher/1
  In1/1 -> Out1/1, Bus Assignment13/2

== system Raider_walk/servos_control/Simulink Function2/Velocity_Publishers/Switch Case Action Subsystem10 ==
  In1 : Inport
  Action Port : ActionPort  ActionType=case
  Blank Message1 : robotlib/Blank Message  SourceLibraryInfo=This block requires Robotics System Toolbox  messageType=std_msgs/Float64  SampleTime=inf
  Bus Assignment1 : BusAssignment  AssignedSignals=Data
  left_ankle_swing_position-Publisher : robotlib/Publish  SourceLibraryInfo=This block requires Robotics System Toolbox  topicSource=Select from ROS network  topic=/raider/l_hip_twist_velocity_controller/command  messageType=std_msgs/Float64  messageQueueLength=1
  Out1 : Outport
  wires:
  Blank Message1/1 -> Bus Assignment1/1
  Bus Assignment1/1 -> left_ankle_swing_position-Publisher/1
  In1/1 -> Out1/1, Bus Assignment1/2

== system Raider_walk/servos_control/Simulink Function2/Velocity_Publishers/Switch Case Action Subsystem11 ==
  In1 : Inport
  Action Port : ActionPort  ActionType=case
  Blank Message1 : robotlib/Blank Message  SourceLibraryInfo=This block requires Robotics System Toolbox  messageType=std_msgs/Float64  SampleTime=inf
  Bus Assignment1 : BusAssignment  AssignedSignals=Data
  left_ankle_swing_position-Publisher : robotlib/Publish  SourceLibraryInfo=This block requires Robotics System Toolbox  topicSource=Select from ROS network  topic=/raider/r_hip_lateral_velocity_controller/command  messageType=std_msgs/Float64  messageQueueLength=1
  Out1 : Outport
  wires:
  Blank Message1/1 -> Bus Assignment1/1
  Bus Assignment1/1 -> left_ankle_swing_position-Publisher/1
  In1/1 -> Out1/1, Bus Assignment1/2

== system Raider_walk/servos_control/Simulink Function2/Velocity_Publishers/Switch Case Action Subsystem12 ==
  In1 : Inport
  Action Port : ActionPort  ActionType=case
  Blank Message1 : robotlib/Blank Message  SourceLibraryInfo=This block requires Robotics System Toolbox  messageType=std_msgs/Float64  SampleTime=inf
  Bus Assignment1 : BusAssignment  AssignedSignals=Data
  left_ankle_swing_position-Publisher : robotlib/Publish  SourceLibraryInfo=This block requires Robotics System Toolbox  topicSource=Select from ROS network  topic=/raider/l_hip_lateral_velocity_controller/command  messageType=std_msgs/Float64  messageQueueLength=1
  Out1 : Outport
  wires:
  Blank Message1/1 -> Bus Assignment1/1
  Bus Assignment1/1 -> left_ankle_swing_position-Publisher/1
  In1/1 -> Out1/1, Bus Assignment1/2

== system Raider_walk/servos_control/Simulink Function2/Velocity_Publishers/Switch Case Action Subsystem13 ==
  In1 : Inport
  Action Port : ActionPort  ActionType=case
  Blank Message1 : robotlib/Blank Message  SourceLibraryInfo=This block requires Robotics System Toolbox  messageType=std_msgs/Float64  SampleTime=inf
  Bus Assignment1 : BusAssignment  AssignedSignals=Data
  left_ankle_swing_position-Publisher : robotlib/Publish  SourceLibraryInfo=This block requires Robotics System Toolbox  topicSource=Select from ROS network  topic=/raider/r_hip_swing_velocity_controller/command  messageType=std_msgs/Float64  messageQueueLength=1
  Out1 : Outport
  wires:
  Blank Message1/1 -> Bus Assignment1/1
  Bus Assignment1/1 -> left_ankle_swing_position-Publisher/1
  In1/1 -> Out1/1, Bus Assignment1/2

== system Raider_walk/servos_control/Simulink Function2/Velocity_Publishers/Switch Case Action Subsystem14 ==
  In1 : Inport
  Action Port : ActionPort  ActionType=case
  Blank Message1 : robotlib/Blank Message  SourceLibraryInfo=This block requires Robotics System Toolbox  messageType=std_msgs/Float64  SampleTime=inf
  Bus Assignment1 : BusAssignment  AssignedSignals=Data
  left_ankle_swing_position-Publisher : robotlib/Publish  SourceLibraryInfo=This block requires Robotics System Toolbox  topicSource=Select from ROS network  topic=/raider/l_hip_swing_velocity_controller/command  messageType=std_msgs/Float64  messageQueueLength=1
  Out1 : Outport
  wires:
  Blank Message1/1 -> Bus Assignment1/1
  Bus Assignment1/1 -> left_ankle_swing_position-Publisher/1
  In1/1 -> Out1/1, Bus Assignment1/2

== system Raider_walk/servos_control/Simulink Function2/Velocity_Publishers/Switch Case Action Subsystem15 ==
  In1 : Inport
  Action Port : ActionPort  ActionType=case
  Blank Message1 : robotlib/Blank Message  SourceLibraryInfo=This block requires Robotics System Toolbox  messageType=std_msgs/Float64  SampleTime=inf
  Bus Assignment1 : BusAssignment  AssignedSignals=Data
  left_ankle_swing_position-Publisher : robotlib/Publish  SourceLibraryInfo=This block requires Robotics System Toolbox  topicSource=Select from ROS network  topic=/raider/r_upper_knee_velocity_controller/command  messageType=std_msgs/Float64  messageQueueLength=1
  Out1 : Outport
  wires:
  Blank Message1/1 -> Bus Assignment1/1
  Bus Assignment1/1 -> left_ankle_swing_position-Publisher/1
  In1/1 -> Out1/1, Bus Assignment1/2

== system Raider_walk/servos_control/Simulink Function2/Velocity_Publishers/Switch Case Action Subsystem16 ==
  In1 : Inport
  Action Port : ActionPort  ActionType=case
  Blank Message1 : robotlib/Blank Message  SourceLibraryInfo=This block requires Robotics System Toolbox  messageType=std_msgs/Float64  SampleTime=inf
  Bus Assignment1 : BusAssignment  AssignedSignals=Data
  left_ankle_swing_position-Publisher : robotlib/Publish  SourceLibraryInfo=This block requires Robotics System Toolbox  topicSource=Select from ROS network  topic=/raider/l_upper_knee_velocity_controller/command  messageType=std_msgs/Float64  messageQueueLength=1
  Out1 : Outport
  wires:
  Blank Message1/1 -> Bus Assignment1/1
  Bus Assignment1/1 -> left_ankle_swing_position-Publisher/1
  In1/1 -> Out1/1, Bus Assignment1/2

== system Raider_walk/servos_control/Simulink Function2/Velocity_Publishers/Switch Case Action Subsystem17 ==
  In1 : Inport
  Action Port : ActionPort  ActionType=case
  Blank Message1 : robotlib/Blank Message  SourceLibraryInfo=This block requires Robotics System Toolbox  messageType=std_msgs/Float64  SampleTime=inf
  Bus Assignment1 : BusAssignment  AssignedSignals=Data
  left_ankle_swing_position-Publisher : robotlib/Publish  SourceLibraryInfo=This block requires Robotics System Toolbox  topicSource=Select from ROS network  topic=/raider/r_ankle_swing_velocity_controller/command  messageType=std_msgs/Float64  messageQueueLength=1
  Out1 : Outport
  wires:
  Blank Message1/1 -> Bus Assignment1/1
  Bus Assignment1/1 -> left_ankle_swing_position-Publisher/1
  In1/1 -> Out1/1, Bus Assignment1/2

== system Raider_walk/servos_control/Simulink Function2/Velocity_Publishers/Switch Case Action Subsystem18 ==
  In1 : Inport
  Action Port : ActionPort  ActionType=case
  Blank Message1 : robotlib/Blank Message  SourceLibraryInfo=This block requires Robotics System Toolbox  messageType=std_msgs/Float64  SampleTime=inf
  Bus Assignment1 : BusAssignment  AssignedSignals=Data
  left_ankle_swing_position-Publisher : robotlib/Publish  SourceLibraryInfo=This block requires Robotics System Toolbox  topicSource=Select from ROS network  topic=/raider/l_ankle_swing_velocity_controller/command  messageType=std_msgs/Float64  messageQueueLength=1
  Out1 : Outport
  wires:
  Blank Message1/1 -> Bus Assignment1/1
  Bus Assignment1/1 -> left_ankle_swing_position-Publisher/1
  In1/1 -> Out1/1, Bus Assignment1/2

== system Raider_walk/servos_control/Simulink Function2/Velocity_Publishers/Switch Case Action Subsystem19 ==
  In1 : Inport
  Action Port : ActionPort  ActionType=case
  Blank Message1 : robotlib/Blank Message  SourceLibraryInfo=This block requires Robotics System Toolbox  messageType=std_msgs/Float64  SampleTime=inf
  Bus Assignment1 : BusAssignment  AssignedSignals=Data
  left_ankle_swing_position-Publisher : robotlib/Publish  SourceLibraryInfo=This block requires Robotics System Toolbox  topicSource=Select from ROS network  topic=/raider/r_ankle_lateral_velocity_controller/command  messageType=std_msgs/Float64  messageQueueLength=1
  Out1 : Outport
  wires:
  Blank Message1/1 -> Bus Assignment1/1
  Bus Assignment1/1 -> left_ankle_swing_position-Publisher/1
  In1/1 -> Out1/1, Bus Assignment1/2

== system Raider_walk/servos_control/Simulink Function2/Velocity_Publishers/Switch Case Action Subsystem2  ==
  In1 : Inport
  Action Port : ActionPort  ActionType=case
  Blank Message4 : robotlib/Blank Message  SourceLibraryInfo=This block requires Robotics System Toolbox  messageType=std_msgs/Float64  SampleTime=inf
  Bus Assignment4 : BusAssignment  AssignedSignals=Data
  left_hip_swing_position-Publisher : robotlib/Publish  SourceLibraryInfo=This block requires Robotics System Toolbox  topicSource=Select from ROS network  topic=/raider/neck_velocity_controller/command  messageType=std_msgs/Float64  messageQueueLength=1
  Out1 : Outport
  wires:
  Blank Message4/1 -> Bus Assignment4/1
  Bus Assignment4/1 -> left_hip_swing_position-Publisher/1
  In1/1 -> Out1/1, Bus Assignment4/2

== system Raider_walk/servos_control/Simulink Function2/Velocity_Publishers/Switch Case Action Subsystem20 ==
  In1 : Inport
  Action Port : ActionPort  ActionType=case
  Blank Message1 : robotlib/Blank Message  SourceLibraryInfo=This block requires Robotics System Toolbox  messageType=std_msgs/Float64  SampleTime=inf
  Bus Assignment1 : BusAssignment  AssignedSignals=Data
  left_ankle_swing_position-Publisher : robotlib/Publish  SourceLibraryInfo=This block requires Robotics System Toolbox  topicSource=Select from ROS network  topic=/raider/l_ankle_lateral_velocity_controller/command  messageType=std_msgs/Float64  messageQueueLength=1
  Out1 : Outport
  wires:
  Blank Message1/1 -> Bus Assignment1/1
  Bus Assignment1/1 -> left_ankle_swing_position-Publisher/1
  In1/1 -> Out1/1, Bus Assignment1/2

== system Raider_walk/servos_control/Simulink Function2/Velocity_Publishers/Switch Case Action Subsystem3  ==
  In1 : Inport
  Action Port : ActionPort  ActionType=case
  Blank Message40 : robotlib/Blank Message  SourceLibraryInfo=This block requires Robotics System Toolbox  messageType=std_msgs/Float64  SampleTime=inf
  Bus Assignment40 : BusAssignment  AssignedSignals=Data
  right_upper_knee_position-Publisher : robotlib/Publish  SourceLibraryInfo=This block requires Robotics System Toolbox  topicSource=Select from ROS network  topic=/raider/r_shoulder_swing_velocity_controller/command  messageType=std_msgs/Float64  messageQueueLength=1
  Out1 : Outport
  wires:
  Blank Message40/1 -> Bus Assignment40/1
  Bus Assignment40/1 -> right_upper_knee_position-Publisher/1
  In1/1 -> Out1/1, Bus Assignment40/2

== system Raider_walk/servos_control/Simulink Function2/Velocity_Publishers/Switch Case Action Subsystem4  ==
  In1 : Inport
  Action Port : ActionPort  ActionType=case
  Blank Message29 : robotlib/Blank Message  SourceLibraryInfo=This block requires Robotics System Toolbox  messageType=std_msgs/Float64  SampleTime=inf
  Bus Assignment29 : BusAssignment  AssignedSignals=Data
  left_upper_knee_position-Publisher : robotlib/Publish  SourceLibraryInfo=This block requires Robotics System Toolbox  topicSource=Select from ROS network  topic=/raider/l_shoulder_swing_velocity_controller/command  messageType=std_msgs/Float64  messageQueueLength=1
  Out1 : Outport
  wires:
  Blank Message29/1 -> Bus Assignment29/1
  Bus Assignment29/1 -> left_upper_knee_position-Publisher/1
  In1/1 -> Out1/1, Bus Assignment29/2

== system Raider_walk/servos_control/Simulink Function2/Velocity_Publishers/Switch Case Action Subsystem5  ==
  In1 : Inport
  Action Port : ActionPort  ActionType=case
  Blank Message10 : robotlib/Blank Message  SourceLibraryInfo=This block requires Robotics System Toolbox  messageType=std_msgs/Float64  SampleTime=inf
  Bus Assignment10 : BusAssignment  AssignedSignals=Data
  right_ankle-swing-Publisher : robotlib/Publish  SourceLibraryInfo=This block requires Robotics System Toolbox  topicSource=Select from ROS network  topic=/raider/r_shoulder_lateral_velocity_controller/command  messageType=std_msgs/Float64  messageQueueLength=1
  Out1 : Outport
  wires:
  Blank Message10/1 -> Bus Assignment10/1
  Bus Assignment10/1 -> right_ankle-swing-Publisher/1
  In1/1 -> Out1/1, Bus Assignment10/2

== system Raider_walk/servos_control/Simulink Function2/Velocity_Publishers/Switch Case Action Subsystem6  ==
  In1 : Inport
  Action Port : ActionPort  ActionType=case
  Blank Message1 : robotlib/Blank Message  SourceLibraryInfo=This block requires Robotics System Toolbox  messageType=std_msgs/Float64  SampleTime=inf
  Bus Assignment1 : BusAssignment  AssignedSignals=Data
  left_ankle_swing_position-Publisher : robotlib/Publish  SourceLibraryInfo=This block requires Robotics System Toolbox  topicSource=Select from ROS network  topic=/raider/l_shoulder_lateral_velocity_controller/command  messageType=std_msgs/Float64  messageQueueLength=1
  Out1 : Outport
  wires:
  In1/1 -> Out1/1, Bus Assignment1/2
  Blank Message1/1 -> Bus Assignment1/1
  Bus Assignment1/1 -> left_ankle_swing_position-Publisher/1

== system Raider_walk/servos_control/Simulink Function2/Velocity_Publishers/Switch Case Action Subsystem7 ==
  In1 : Inport
  Action Port : ActionPort  ActionType=case
  Blank Message1 : robotlib/Blank Message  SourceLibraryInfo=This block requires Robotics System Toolbox  messageType=std_msgs/Float64  SampleTime=inf
  Bus Assignment1 : BusAssignment  AssignedSignals=Data
  left_ankle_swing_position-Publisher : robotlib/Publish  SourceLibraryInfo=This block requires Robotics System Toolbox  topicSource=Select from ROS network  topic=/raider/r_elbow_velocity_controller/command  messageType=std_msgs/Float64  messageQueueLength=1
  Out1 : Outport
  wires:
  Blank Message1/1 -> Bus Assignment1/1
  Bus Assignment1/1 -> left_ankle_swing_position-Publisher/1
  In1/1 -> Out1/1, Bus Assignment1/2

== system Raider_walk/servos_control/Simulink Function2/Velocity_Publishers/Switch Case Action Subsystem8 ==
  In1 : Inport
  Action Port : ActionPort  ActionType=case
  Blank Message1 : robotlib/Blank Message  SourceLibraryInfo=This block requires Robotics System Toolbox  messageType=std_msgs/Float64  SampleTime=inf
  Bus Assignment1 : BusAssignment  AssignedSignals=Data
  left_ankle_swing_position-Publisher : robotlib/Publish  SourceLibraryInfo=This block requires Robotics System Toolbox  topicSource=Select from ROS network  topic=/raider/l_elbow_velocity_controller/command  messageType=std_msgs/Float64  messageQueueLength=1
  Out1 : Outport
  wires:
  Blank Message1/1 -> Bus Assignment1/1
  Bus Assignment1/1 -> left_ankle_swing_position-Publisher/1
  In1/1 -> Out1/1, Bus Assignment1/2

== system Raider_walk/servos_control/Simulink Function2/Velocity_Publishers/Switch Case Action Subsystem9 ==
  In1 : Inport
  Action Port : ActionPort  ActionType=case
  Blank Message1 : robotlib/Blank Message  SourceLibraryInfo=This block requires Robotics System Toolbox  messageType=std_msgs/Float64  SampleTime=inf
  Bus Assignment1 : BusAssignment  AssignedSignals=Data
  left_ankle_swing_position-Publisher : robotlib/Publish  SourceLibraryInfo=This block requires Robotics System Toolbox  topicSource=Select from ROS network  topic=/raider/r_hip_twist_velocity_controller/command  messageType=std_msgs/Float64  messageQueueLength=1
  Out1 : Outport
  wires:
  Blank Message1/1 -> Bus Assignment1/1
  Bus Assignment1/1 -> left_ankle_swing_position-Publisher/1
  In1/1 -> Out1/1, Bus Assignment1/2

== matlab function Raider_walk/servos_control/MATLAB Function ==
  data: t input; targetPosition data_store_memory; currentPosition data_store_memory
function move_joints(t)

% It takes as input the time in seconds (typical values are between 0.5 and
% 0.1 seconds) in which the joints should reach new postions. It calls the
% publish_Position function in a loop with all the values of the targetPosition(20)
% array. Also, it computes the absolute value of the difference between the
% currentPosition(20) and targetPosition(20) for all joints and divides it into the
% time specified to send different velocity commands to each joint calling the
% publishVelocity function, so that they reach positions at the same time and make
% simultaneous motions and the robot inertial disturbance is lower


global currentPosition;
global targetPosition;



for idx=1:20
    publishPosition(idx, targetPosition(idx));
    publishVelocity(idx, abs(targetPosition(idx)-currentPosition(idx))/t);

end



delay(t);


updateCurrentPosition();
